simulink model "roll_angle_design_step"  (R2019b)
settings: Solver=FixedStepAuto  StartTime=0.0  StopTime=step_sim_time  FixedStep=1/step_sim_freq  RelTol=1e-3
values from neighbouring files (symbols this model uses):
  disturb = 1    [rootlocus.m]
  disturb_time = 20    [rootlocus.m]
  Kp_ra = 3    [rootlocus.m]
  step_time = 0    [rootlocus.m]
settings Model: Creator=francois  LastModifiedBy=francois

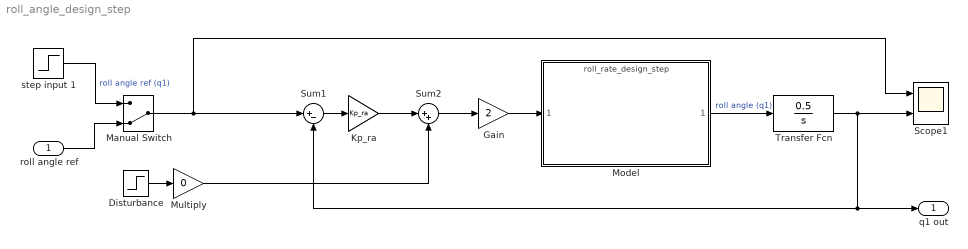
== system roll_angle_design_step ==
  "roll angle ref " : Inport
  "Disturbance " : Step  Time=disturb_time  After=disturb  SampleTime=0
  Gain : Gain  Gain=2
  Kp_ra : Gain  Gain=Kp_ra
  Manual Switch : ManualSwitch  CurrentSetting=0
  Model : ModelReference  ModelNameDialog=roll_rate_design_step.slx  SimulationMode=Normal  ModelReferenceVersion=1.4
  Multiply : Gain  Gain=0
  Scope1 : Scope  NumInputPorts=2
  Sum1 : Sum  Inputs=|+-
  Sum2 : Sum  Inputs=|++
  Transfer Fcn : TransferFcn  Numerator=[0.5]  Denominator=[1 0]
  step input 1 : Step  Time=step_time  SampleTime=0
  "q1 out " : Outport  SignalName=q1 out
  wires:
  Model/1 -> Transfer Fcn/1  "roll angle (q1)"
  "Disturbance "/1 -> Multiply/1
  Gain/1 -> Model/1
  Multiply/1 -> Sum2/2
  Transfer Fcn/1 -> "q1 out "/1, Sum1/2, Scope1/2
  Kp_ra/1 -> Sum2/1
  Sum1/1 -> Kp_ra/1
  Sum2/1 -> Gain/1
  Manual Switch/1 -> Scope1/1, Sum1/1
  step input 1/1 -> Manual Switch/1  "roll angle ref (q1)"
  "roll angle ref "/1 -> Manual Switch/2
